simulink model "bldc_speed_ctrl"  (R2020a)
settings: Solver=VariableStepAuto  StartTime=0.0  StopTime=10.0  RelTol=1e-3
model workspace (MAT data in the model file):
  Kd = 0.0001851
  Ke = 0.0275
  Ki = 1350.074
  Kp = 12
  Kt = 0.0275
settings Model: Creator=Shubham  LastModifiedBy=Shubham

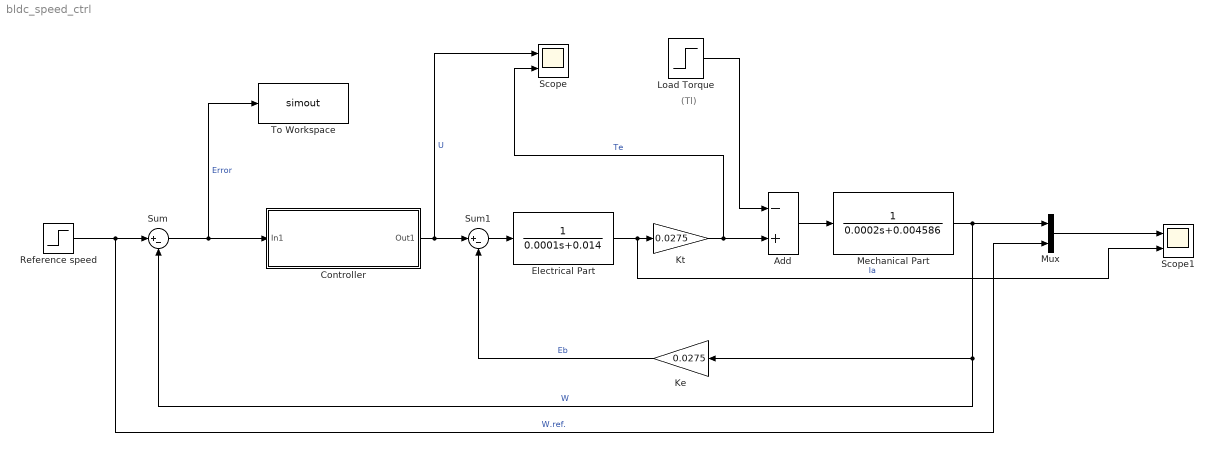
== system bldc_speed_ctrl ==
  note: (Tl)
  Add : Sum  Inputs=-+
  Controller : Subsystem
  Electrical Part : TransferFcn  Denominator=[0.0001 0.014]
  Ke : Gain  Gain=0.0275
  Kt : Gain  Gain=0.0275
  Load Torque : Step  Time=0.1  After=10  SampleTime=0
  Mechanical Part : TransferFcn  Denominator=[0.0002 0.004586]
  Mux : Mux  Inputs=2
  Reference speed : Step  After=1500  SampleTime=0
  Scope : Scope  NumInputPorts=2
  Scope1 : Scope  NumInputPorts=2
  Sum : Sum  Inputs=|+-
  Sum1 : Sum  Inputs=|+-
  To Workspace : ToWorkspace  VariableName=simout  SaveFormat=Timeseries  SampleTime=-1
  wires:
  Reference speed/1 -> Mux/2, Sum/1  "W.ref."
  Sum/1 -> To Workspace/1, Controller/1(In1)  "Error"
  Controller/1(Out1) -> Scope/1, Sum1/1  "U"
  Kt/1 -> Scope/2, Add/2  "Te"
  Sum1/1 -> Electrical Part/1
  Electrical Part/1 -> Scope1/2, Kt/1  "Ia"
  Load Torque/1 -> Add/1
  Mux/1 -> Scope1/1
  Add/1 -> Mechanical Part/1
  Ke/1 -> Sum1/2  "Eb"
  Mechanical Part/1 -> Sum/2, Ke/1, Mux/1  "W"

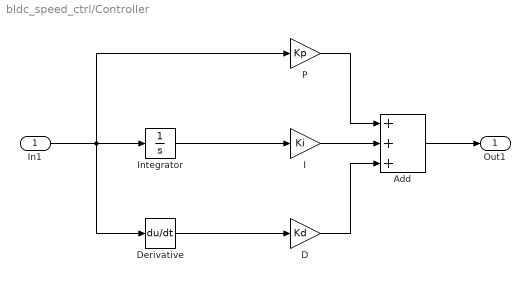
== system bldc_speed_ctrl/Controller ==
  In1 : Inport
  Add : Sum  Inputs=+++
  D : Gain  Gain=Kd
  Derivative : Derivative
  I : Gain  Gain=Ki
  Integrator : Integrator
  P : Gain  Gain=Kp
  Out1 : Outport
  wires:
  In1/1 -> Derivative/1, P/1, Integrator/1
  Integrator/1 -> I/1
  I/1 -> Add/2
  Add/1 -> Out1/1
  P/1 -> Add/1
  D/1 -> Add/3
  Derivative/1 -> D/1
